simulink model "SF001A_Assi"  (R2013b)
settings: Solver=FixedStepDiscrete  StartTime=0.0  StopTime=1  FixedStep=.002  RelTol=1e-3
values from neighbouring files (symbols this model uses):
  FLTINJ_ASSI_ASSICMDBAS = DataDict.Constant    [SF001A_Assi_DataDict.m]
libraries: FixdToFloat x4, FloatToFixd x4, BilnrIntrpnMplX x3, NxtrLim x2, NxtrAbslt x1, NxtrMath x1, LnrIntrpn x1, NxtrSign x1, simulink x1
settings Model: Creator=lzz0tm  LastModifiedBy=HZQ8V7
settings DataIOCC: LimitDataPoints=off  SaveFormat=Structure  ReturnWorkspaceOutputs=on
settings OptimizationCC: BlockReduction=off  InlineParams=on  ZeroExternalMemoryAtStartup=off  ZeroInternalMemoryAtStartup=off  OptimizeModelRefInitCode=on  LifeSpan=1
settings DebuggingCC: SignalInfNanChecking=error  SignalRangeChecking=warning  UnderspecifiedInitializationDetection=Simplified  SolverPrmCheckMsg=error  InheritedTsInSrcMsg=error  DiscreteInheritContinuousMsg=error  SingleTaskRateTransMsg=error  TasksWithSamePriorityMsg=error  SigSpecEnsureSampleTimeMsg=error  CheckMatrixSingularityMsg=error  IntegerOverflowMsg=error  ParameterUnderflowMsg=error  ParameterPrecisionLossMsg=error  ParameterTunabilityLossMsg=error  FixptConstUnderflowMsg=warning  FixptConstOverflowMsg=warning  VectorMatrixConversionMsg=error  SignalLabelMismatchMsg=error  UnconnectedInputMsg=error  UnconnectedOutputMsg=error  UnconnectedLineMsg=error  SFcnCompatibilityMsg=error  UniqueDataStoreMsg=warning  BusObjectLabelMismatch=error  RootOutportRequireBusObject=error  AssertControl=DisableAll  ModelReferenceIOMsg=error  ModelReferenceVersionMismatchMessage=warning  ModelReferenceIOMismatchMessage=error  ModelReferenceCSMismatchMessage=warning  ModelReferenceDataLoggingMessage=error  StateNameClashWarn=warning  StrictBusMsg=ErrorOnBusTreatedAsVector  NonBusSignalsTreatedAsBus=error  SFUnexpectedBacktrackingDiag=error  SFInvalidInputDataAccessInChartInitDiag=error  SFNoUnconditionalDefaultTransitionDiag=error  SFTransitionOutsideNaturalParentDiag=error  SFUnconditionalTransitionShadowingDiag=error  SFUndirectedBroadcastEventsDiag=error
settings ModelReferenceCC: ModelReferenceNumInstancesAllowed=Single
settings RTWCC: SystemTargetFile=autosar.tlc  GenCodeOnly=on  TemplateMakefile=ert_default_tmf  Description=AUTOSAR  GenerateReport=on  ProcessScript=autosar_make_rtw_hook  LaunchReport=on
settings CodeAppCC: GenerateComments=off  IgnoreCustomStorageClasses=off  CustomSymbolStrType=$N$R$M  CustomSymbolStrBlkIO=$N$M  SimulinkBlockComments=off
settings STFCustomTargetCC: ParMdlRefBuildCompliant=on  CompOptLevelCompliant=on  IncludeMdlTerminateFcn=off  CombineOutputUpdateFcns=on  SuppressErrorStatus=on  ERTFirstTimeCompliant=on  ERTCustomFileBanners=on  SupportNonFinite=off  SupportComplex=off  SupportContinuousTime=off  SupportNonInlinedSFcns=off  MATLABClassNameForMDSCustomization=Simulink.SoftwareTarget.ERTCustomization  AutosarCompliant=on  GRTInterface=off  SystemTargetFile=autosar.tlc
settings ERTTargetCC: CodeReplacementLibrary=ANSI_C  ConcurrentExecutionCompliant=off  IncludeMdlTerminateFcn=off  SuppressErrorStatus=on  SupportNonFinite=off  SupportComplex=off  ModelStepFunctionPrototypeControlCompliant=off  CPPClassGenCompliant=off  AutosarCompliant=on  InlinedParameterPlacement=NonHierarchical  ERTCustomFileTemplate=example_file_process.tlc  EnableUserReplacementTypes=on

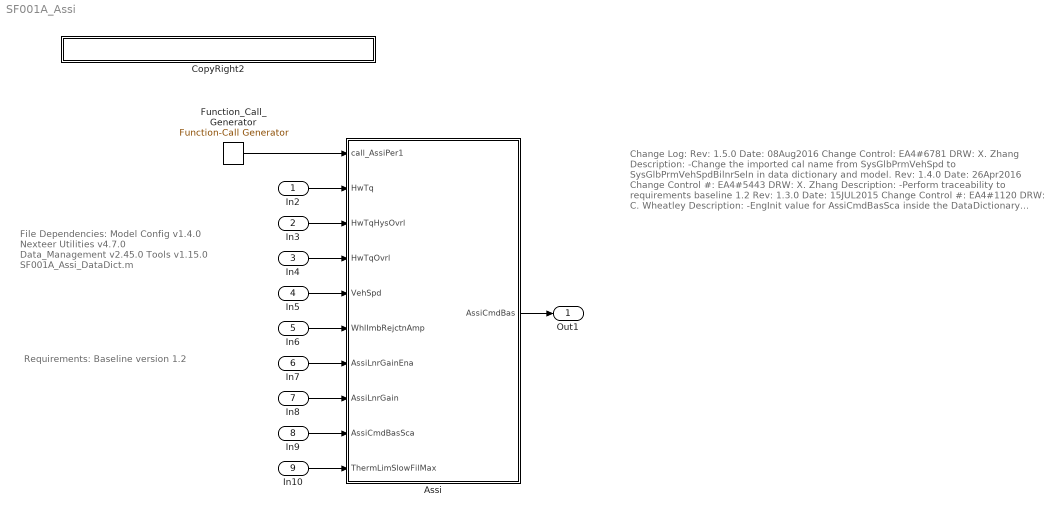
== system SF001A_Assi ==
  note: File Dependencies:
      |
      | Model Config v1.4.0
      | Nexteer Utilities v4.7.0
      | Data_Management v2.45.0
      | Tools v1.15.0
      | SF001A_Assi_DataDict.m
  note: Change Log:
      |
      | Rev: 1.5.0
      | Date: 08Aug2016
      | Change Control: EA4#6781
      | DRW: X. Zhang
      | Description:
      | -Change the imported cal name from SysGlbPrmVehSpd
      | to SysGlbPrmVehSpdBilnrSeln in data dictionary and model.
      |
      |
      | Rev: 1.4.0
      | Date: 26Apr2016
      | Change Control #: EA4#5443
      | DRW: X. Zhang
      | Description:
      | -Perform traceability to requirements baseline 1.2
      |
      | Rev: 1.3.0
      | Date: 15JUL2015
      | Change Control #: EA4#1120
      | DRW: C. Wheatley
      | Description:
      | -EngInit value for AssiCmdBasSca inside the
      |   DataDictionary changed to 1
      |
      | Rev: 1.2.0
      | Date: 09JUN2015
      | Change Control #: EA4#729
      | DRW: C. Wheatley
      | Description:
      | - Fault Injection mistake corrected in the model
      | - Variable names in DataDictionary changed to
      |    comply with AutoSar
      | - LongName and Description fixes in the
      |    DataDictionary
      | - Calibration settings corrected in DataDictionary
      | - Boolean If statement in model adjusted for
      |    readability
      | - Blend now using EA4 block
      | - Naming consistency in the model
      |
      | Rev: 1.1.0
      | Date: 28MAY2015
      | Change Control #: EA4#675
      | DRW: C. Wheatley
      | Description:
      | - Updated changes to the DataDictionary values
      | - Model updated to use global parameters
      |
      | Rev: 1.0.0
      | Date: 28APR2015
      | Change Control #: EA4#513
      | DRW: Wheatley
      | Description:
      | Initial EA4 Release
  note: Requirements: Baseline version 1.2
  In2 : Inport
  In3 : Inport  Port=2
  In4 : Inport  Port=3
  In5 : Inport  Port=4
  In6 : Inport  Port=5
  In7 : Inport  Port=6
  In8 : Inport  Port=7
  In9 : Inport  Port=8
  In10 : Inport  Port=9
  Assi : Subsystem
  CopyRight2 : Subsystem  Description=|  mask(Copyright Information){none=on}
      | Copyright info block.                                               
      |                                                                     
      | Place copyright information at the top of every subsystem in design.
      mask prompts: none "No parameters"
      mask help: Place copyright information at the top of every subsystem in design.
      mask Display:
      | NxtrConf = 'Nexteer Confidential';
      | 
      | sys = bdroot; %handle for the current model ("system")
      | first = get_param(sys,'Created');
      | first = first(end-3:end);  %year is last four digits
      | 
      | last = get_param(sys,'LastModifiedDate');
      | if isempty(last)
      |     last = datestr(now,'yyyy');
      | else
      |     last = last(end-3:end);
      | end
      | 
      | if strcmp(first,last)
      |     fprintf('%s -- Copyright %s Nexteer',NxtrConf,first)
      | else
      |     fprintf('%s -- %s%s- %s Nexteer',NxtrConf,char(169),first,last)
      | end
  Function_Call_Generator : simulink/Ports & Subsystems/Function-Call Generator  sample_time=1  numberOfIterations=1
  Out1 : Outport
  wires:
  In4/1 -> Assi/4(HwTqOvrl)
  In3/1 -> Assi/3(HwTqHysOvrl)
  In2/1 -> Assi/2(HwTq)
  Function_Call_Generator/1 -> Assi/1("call_AssiPer1 ")
  In5/1 -> Assi/5(VehSpd)
  In6/1 -> Assi/6(WhlImbRejctnAmp)
  In7/1 -> Assi/7(AssiLnrGainEna)
  In8/1 -> Assi/8(AssiLnrGain)
  In9/1 -> Assi/9(AssiCmdBasSca)
  In10/1 -> Assi/10(ThermLimSlowFilMax)
  Assi/1(AssiCmdBas) -> Out1/1

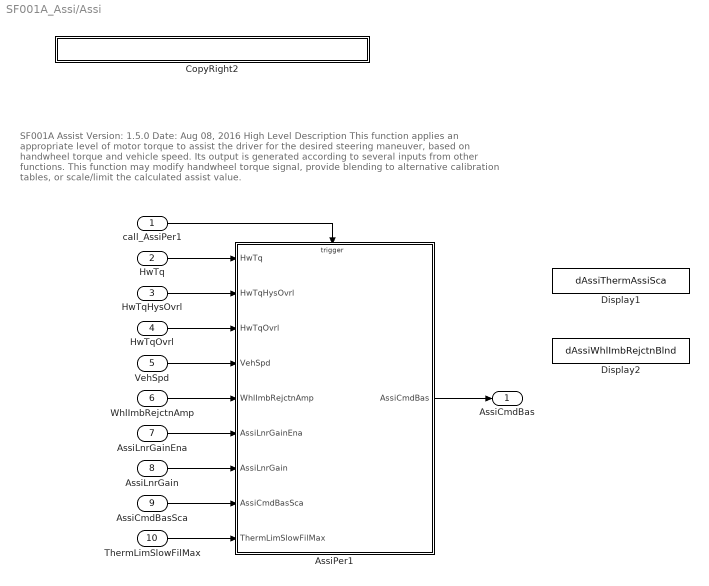
== system SF001A_Assi/Assi ==
  note: SF001A Assist                                                                                  Version:  1.5.0         Date:  Aug 08, 2016
      |  High Level Description
      |
      | This function applies an appropriate level of motor torque to assist the driver for the desired steering maneuver,
      | based on handwheel torque and vehicle speed. Its output is generated according to several inputs from other functions.
      | This function may modify handwheel torque signal, provide blending to alternative calibration tables, or scale/limit the calculated assist value.
  "call_AssiPer1 " : Inport
  HwTq : Inport  RequirementInfo={'linktype_rmi_doors' '0000a523 (/E-STEER Core/SubSystem Specifications/Application Functions/SF001A Assist)' '#SF001A_565' 'true' 'REQ: SF001A_565' '' } %GIDa_df1c7e41_35b1_4231_b879_3ebd4c9f1c76  Port=2  PortDimensions=1
  HwTqHysOvrl : Inport  RequirementInfo={'linktype_rmi_doors' '0000a523 (/E-STEER Core/SubSystem Specifications/Application Functions/SF001A Assist)' '#SF001A_566' 'true' 'REQ: SF001A_566' '' } %GIDa_321f90ce_d978_4ab3_928c_b38d2719cd45  Port=3
  HwTqOvrl : Inport  RequirementInfo={'linktype_rmi_doors' '0000a523 (/E-STEER Core/SubSystem Specifications/Application Functions/SF001A Assist)' '#SF001A_566' 'true' 'REQ: SF001A_566' '' } %GIDa_7605816b_6934_4ac2_b90b_cbcd1f03215b  Port=4
  VehSpd : Inport  RequirementInfo={'linktype_rmi_doors' '0000a523 (/E-STEER Core/SubSystem Specifications/Application Functions/SF001A Assist)' '#SF001A_566' 'true' 'REQ: SF001A_566' '' } %GIDa_a7343de8_f548_4ff5_81a9_3f5168f89c4e  Port=5
  WhlImbRejctnAmp : Inport  RequirementInfo={'linktype_rmi_doors' '0000a523 (/E-STEER Core/SubSystem Specifications/Application Functions/SF001A Assist)' '#SF001A_569' 'true' 'REQ: SF001A_569' '' } %GIDa_b330648f_a269_46fd_8bc1_16a6ad0b258f  Port=6
  AssiLnrGainEna : Inport  RequirementInfo={'linktype_rmi_doors' '0000a523 (/E-STEER Core/SubSystem Specifications/Application Functions/SF001A Assist)' '#SF001A_570' 'true' 'REQ: SF001A_570' '' } %GIDa_c83e3dc0_0b95_4f73_8c8d_f554ad8bd146  Port=7
  AssiLnrGain : Inport  RequirementInfo={'linktype_rmi_doors' '0000a523 (/E-STEER Core/SubSystem Specifications/Application Functions/SF001A Assist)' '#SF001A_571' 'true' 'REQ: SF001A_571' '' } %GIDa_7839c29a_d675_4409_929b_04df3bfe5379  Port=8
  AssiCmdBasSca : Inport  RequirementInfo={'linktype_rmi_doors' '0000a523 (/E-STEER Core/SubSystem Specifications/Application Functions/SF001A Assist)' '#SF001A_572' 'true' 'REQ: SF001A_572' '' } %GIDa_8964cba7_7b16_46dc_9776_5743dbedca3e  Port=9
  ThermLimSlowFilMax : Inport  RequirementInfo={'linktype_rmi_doors' '0000a523 (/E-STEER Core/SubSystem Specifications/Application Functions/SF001A Assist)' '#SF001A_573' 'true' 'REQ: SF001A_573' '' } %GIDa_45ade21b_63ba_460c_b3cc_31c25871d07a  Port=10
  AssiPer1 : Subsystem
  CopyRight2 : Subsystem  Description=|  mask(Copyright Information){none=on}
      | Copyright info block.                                               
      |                                                                     
      | Place copyright information at the top of every subsystem in design.
      mask prompts: none "No parameters"
      mask help: Place copyright information at the top of every subsystem in design.
      mask Display:
      | NxtrConf = 'Nexteer Confidential';
      | 
      | sys = bdroot; %handle for the current model ("system")
      | first = get_param(sys,'Created');
      | first = first(end-3:end);  %year is last four digits
      | 
      | last = get_param(sys,'LastModifiedDate');
      | if isempty(last)
      |     last = datestr(now,'yyyy');
      | else
      |     last = last(end-3:end);
      | end
      | 
      | if strcmp(first,last)
      |     fprintf('%s -- Copyright %s Nexteer',NxtrConf,first)
      | else
      |     fprintf('%s -- %s%s- %s Nexteer',NxtrConf,char(169),first,last)
      | end
  Display1 : DataStoreMemory  DataStoreName=dAssiThermAssiSca  ReadBeforeWriteMsg=warning  WriteAfterWriteMsg=warning  WriteAfterReadMsg=warning  StateMustResolveToSignalObject=on
  Display2 : DataStoreMemory  DataStoreName=dAssiWhlImbRejctnBlnd  ReadBeforeWriteMsg=warning  WriteAfterWriteMsg=warning  WriteAfterReadMsg=warning  StateMustResolveToSignalObject=on
  AssiCmdBas : Outport  RequirementInfo={'linktype_rmi_doors' '0000a523 (/E-STEER Core/SubSystem Specifications/Application Functions/SF001A Assist)' '#SF001A_573' 'true' 'REQ: SF001A_573' '' } %GIDa_c295ac1d_a023_4c71_a7e9_db668cfce82d
  wires:
  "call_AssiPer1 "/1 -> AssiPer1/Trigger
  AssiCmdBasSca/1 -> AssiPer1/8(AssiCmdBasSca)
  ThermLimSlowFilMax/1 -> AssiPer1/9(ThermLimSlowFilMax)
  HwTqOvrl/1 -> AssiPer1/3(HwTqOvrl)
  HwTqHysOvrl/1 -> AssiPer1/2(HwTqHysOvrl)
  HwTq/1 -> AssiPer1/1(HwTq)
  AssiLnrGain/1 -> AssiPer1/7(AssiLnrGain)
  WhlImbRejctnAmp/1 -> AssiPer1/5(WhlImbRejctnAmp)
  AssiPer1/1(AssiCmdBas) -> AssiCmdBas/1
  AssiLnrGainEna/1 -> AssiPer1/6(AssiLnrGainEna)
  VehSpd/1 -> AssiPer1/4(VehSpd)

== system SF001A_Assi/CopyRight2 ==

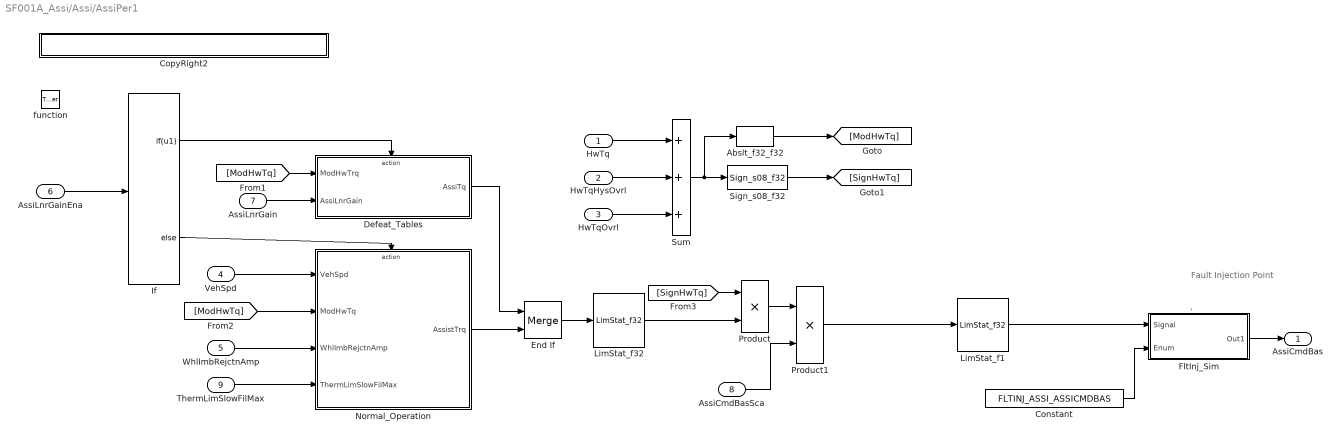
== system SF001A_Assi/Assi/AssiPer1 ==
  note: ,
  note: Fault
      | Injection
      | Point
  HwTq : Inport  RequirementInfo={'linktype_rmi_doors' '0000a523 (/E-STEER Core/SubSystem Specifications/Application Functions/SF001A Assist)' '#SF001A_565' 'true' 'REQ: SF001A_565' '' } %GIDa_4c532047_88a3_4a73_b7dd_64dbcaaed348  PortDimensions=1
  HwTqHysOvrl : Inport  RequirementInfo={'linktype_rmi_doors' '0000a523 (/E-STEER Core/SubSystem Specifications/Application Functions/SF001A Assist)' '#SF001A_565' 'true' 'REQ: SF001A_565' '' } %GIDa_a6de7906_5536_4fc7_b71a_7e4fd7338639  Port=2
  HwTqOvrl : Inport  RequirementInfo={'linktype_rmi_doors' '0000a523 (/E-STEER Core/SubSystem Specifications/Application Functions/SF001A Assist)' '#SF001A_565' 'true' 'REQ: SF001A_565' '' } %GIDa_743579df_9034_4b45_9394_2ab6ce07898f  Port=3
  VehSpd : Inport  Port=4
  WhlImbRejctnAmp : Inport  Port=5
  AssiLnrGainEna : Inport  Port=6
  AssiLnrGain : Inport  Port=7
  AssiCmdBasSca : Inport  RequirementInfo={'linktype_rmi_doors' '0000a523 (/E-STEER Core/SubSystem Specifications/Application Functions/SF001A Assist)' '#SF001A_54' 'true' 'REQ: SF001A_54' '' } %GIDa_4f99cdde_4310_4043_a572_c6e40ed4e5b1  Port=8
  ThermLimSlowFilMax : Inport  Port=9
  function : TriggerPort  TriggerType=function-call  PortDimensions=1
  Abslt_f32_f32 : NxtrAbslt/Abslt_f32_f32  RequirementInfo={'linktype_rmi_doors' '0000a523 (/E-STEER Core/SubSystem Specifications/Application Functions/SF001A Assist)' '#SF001A_565' 'true' 'REQ: SF001A_565' '' } %GIDa_e7f45768_8990_4d11_92fe_2addd2fec813  SFunctionSpec=single y1 = Abslt_f32_f32(single u1)
  Constant : Constant  Value=FLTINJ_ASSI_ASSICMDBAS
  CopyRight2 : Subsystem  Description=|  mask(Copyright Information){none=on}
      | Copyright info block.                                               
      |                                                                     
      | Place copyright information at the top of every subsystem in design.
      mask prompts: none "No parameters"
      mask help: Place copyright information at the top of every subsystem in design.
      mask Display:
      | NxtrConf = 'Nexteer Confidential';
      | 
      | sys = bdroot; %handle for the current model ("system")
      | first = get_param(sys,'Created');
      | first = first(end-3:end);  %year is last four digits
      | 
      | last = get_param(sys,'LastModifiedDate');
      | if isempty(last)
      |     last = datestr(now,'yyyy');
      | else
      |     last = last(end-3:end);
      | end
      | 
      | if strcmp(first,last)
      |     fprintf('%s -- Copyright %s Nexteer',NxtrConf,first)
      | else
      |     fprintf('%s -- %s%s- %s Nexteer',NxtrConf,char(169),first,last)
      | end
  Defeat_Tables : Subsystem  RequirementInfo={} %GIDa_71bd2140_2601_481a_a962_dd66954b4836  TreatAsAtomicUnit=on
  End If : Merge
  FltInj_Sim : Subsystem  RequirementInfo={} %GIDa_e6d32a6b_110d_43d3_bf1f_53358b823df8  TreatAsAtomicUnit=on  VariantControl=FltInj_sim  mask(Fault_Injection){}
      mask help: Fault Injection is a simulation only block for EA4 programs.
  If : If  RequirementInfo={'linktype_rmi_doors' '0000a523 (/E-STEER Core/SubSystem Specifications/Application Functions/SF001A Assist)' '#SF001A_584' 'true' 'REQ: SF001A_584' '' ; 'linktype_rmi_doors' '0000a523 (/E-STEER Core/SubSystem Specifications/Application Functions/SF001A Assist)' '#SF001A_586' 'true' 'REQ: SF001A_586' '' } %GIDa_38834bf7_fb6d_4a7f_939f_eb78c484652c  IfExpression=u1
  LimStat_f1 : NxtrLim/LimStat_f32  RequirementInfo={'linktype_rmi_doors' '0000a523 (/E-STEER Core/SubSystem Specifications/Application Functions/SF001A Assist)' '#SF001A_596' 'true' 'REQ: SF001A_596' '' } %GIDa_3652e6d3_c985_43e4_abfc_04d6d52d1687  LoLim=SYSGLBPRM_MOTTQCMDLOLIM_MOTNWTMTR_F32  HiLim=SYSGLBPRM_MOTTQCMDHILIM_MOTNWTMTR_F32
      settings: AttributesFormatString=|
      | Low Limit: %<LoLim>
      | High Limit: %<HiLim>
  LimStat_f32 : NxtrLim/LimStat_f32  RequirementInfo={'linktype_rmi_doors' '0000a523 (/E-STEER Core/SubSystem Specifications/Application Functions/SF001A Assist)' '#SF001A_593' 'true' 'REQ: SF001A_593' '' } %GIDa_e2683ff8_6aed_4c9d_9aec_fac7f0f7d52d  LoLim=ASSITQSFTYLIM_MOTNWTMTR_F32  HiLim=SYSGLBPRM_MOTTQCMDHILIM_MOTNWTMTR_F32
      settings: AttributesFormatString=|
      | Low Limit: %<LoLim>
      | High Limit: %<HiLim>
  Normal_Operation : Subsystem  RequirementInfo={} %GIDa_a17e3b27_231d_4f75_8813_4f769b98bbc6  TreatAsAtomicUnit=on
  Product : Product  RequirementInfo={'linktype_rmi_doors' '0000a523 (/E-STEER Core/SubSystem Specifications/Application Functions/SF001A Assist)' '#SF001A_595' 'true' 'REQ: SF001A_595' '' } %GIDa_1e6d8c6c_cd19_4240_97f1_349498f31d5f  RndMeth=Zero
  Product1 : Product  RequirementInfo={'linktype_rmi_doors' '0000a523 (/E-STEER Core/SubSystem Specifications/Application Functions/SF001A Assist)' '#SF001A_595' 'true' 'REQ: SF001A_595' '' } %GIDa_d1996e46_02c0_494a_8107_cfbf4a1e6ec3  RndMeth=Zero
  Sign_s08_f32 : NxtrSign/Sign_s08_f32  RequirementInfo={} %GIDa_76fc9d16_9ca3_42b5_94b3_bead8e1e389b  SFunctionSpec=int8 y1 = Sign_s08_f32(single u1)
  Sum : Sum  RequirementInfo={'linktype_rmi_doors' '0000a523 (/E-STEER Core/SubSystem Specifications/Application Functions/SF001A Assist)' '#SF001A_581' 'true' 'REQ: SF001A_581' '' } %GIDa_5bf640b0_a2a0_4a1b_859a_3210dc25e735  Inputs=+++
  AssiCmdBas : Outport  RequirementInfo={} %GIDa_2c9965c4_fb6f_4fb8_804f_ca6f7a7ece36
  wires:
  Product1/1 -> LimStat_f1/1
  Abslt_f32_f32/1 -> [ModHwTq]
  [SignHwTq] -> Product/1
  Sum/1 -> Sign_s08_f32/1, Abslt_f32_f32/1
  HwTq/1 -> Sum/1
  HwTqHysOvrl/1 -> Sum/2
  HwTqOvrl/1 -> Sum/3
  AssiLnrGainEna/1 -> If/1
  If/1 -> Defeat_Tables/Action
  If/2 -> Normal_Operation/Action
  [ModHwTq] -> Defeat_Tables/1(ModHwTrq)
  [ModHwTq] -> Normal_Operation/2(ModHwTq)
  WhlImbRejctnAmp/1 -> Normal_Operation/3(WhlImbRejctnAmp)
  VehSpd/1 -> Normal_Operation/1(VehSpd)
  Defeat_Tables/1(AssiTq) -> End If/1
  Normal_Operation/1(AssistTrq) -> End If/2
  AssiLnrGain/1 -> Defeat_Tables/2(AssiLnrGain)
  Product/1 -> Product1/1
  ThermLimSlowFilMax/1 -> Normal_Operation/4(ThermLimSlowFilMax)
  AssiCmdBasSca/1 -> Product1/2
  Sign_s08_f32/1 -> [SignHwTq]
  End If/1 -> LimStat_f32/1
  LimStat_f32/1 -> Product/2
  LimStat_f1/1 -> FltInj_Sim/1(Signal)
  Constant/1 -> FltInj_Sim/2(Enum)
  FltInj_Sim/1(Out1) -> AssiCmdBas/1

== system SF001A_Assi/Assi/CopyRight2 ==

== system SF001A_Assi/Assi/AssiPer1/CopyRight2 ==

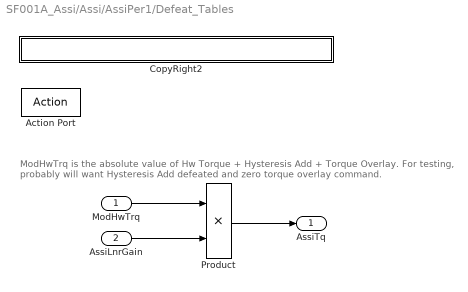
== system SF001A_Assi/Assi/AssiPer1/Defeat_Tables ==
  note: ModHwTrq is the absolute value of Hw Torque  +  Hysteresis Add  +  Torque Overlay.
      | For testing, probably will want Hysteresis Add defeated and zero torque overlay command.
  ModHwTrq : Inport
  AssiLnrGain : Inport  Port=2
  Action Port : ActionPort  ActionType=then
  CopyRight2 : Subsystem  Description=|  mask(Copyright Information){none=on}
      | Copyright info block.                                               
      |                                                                     
      | Place copyright information at the top of every subsystem in design.
      mask prompts: none "No parameters"
      mask help: Place copyright information at the top of every subsystem in design.
      mask Display:
      | NxtrConf = 'Nexteer Confidential';
      | 
      | sys = bdroot; %handle for the current model ("system")
      | first = get_param(sys,'Created');
      | first = first(end-3:end);  %year is last four digits
      | 
      | last = get_param(sys,'LastModifiedDate');
      | if isempty(last)
      |     last = datestr(now,'yyyy');
      | else
      |     last = last(end-3:end);
      | end
      | 
      | if strcmp(first,last)
      |     fprintf('%s -- Copyright %s Nexteer',NxtrConf,first)
      | else
      |     fprintf('%s -- %s%s- %s Nexteer',NxtrConf,char(169),first,last)
      | end
  Product : Product  RequirementInfo={} %GIDa_47c2f9d0_cfe8_45f5_bf6e_658d390a0821  RndMeth=Zero
  AssiTq : Outport  RequirementInfo={'linktype_rmi_doors' '0000a523 (/E-STEER Core/SubSystem Specifications/Application Functions/SF001A Assist)' '#SF001A_585' 'true' 'REQ: SF001A_585' '' } %GIDa_b2d1d4b3_a613_4d35_bc31_c1b4db410c70
  wires:
  ModHwTrq/1 -> Product/1
  Product/1 -> AssiTq/1
  AssiLnrGain/1 -> Product/2

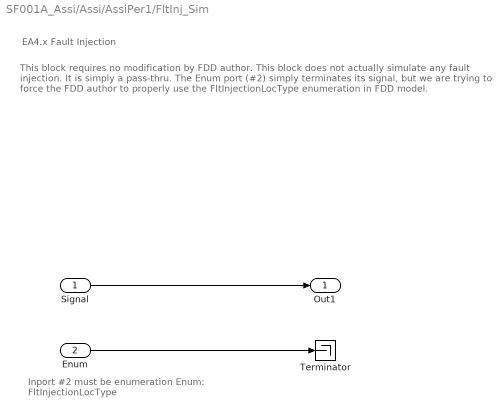
== system SF001A_Assi/Assi/AssiPer1/FltInj_Sim ==
  note: Inport #2 must be enumeration
      | Enum: FltInjectionLocType
  note: EA4.x Fault Injection
  note: This block requires no modification by FDD author.
      |
      | This block does not actually simulate any fault injection.  It is simply a pass-thru.
      |
      | The Enum port (#2) simply terminates its signal, but we are trying to force the FDD author
      | to properly use the FltInjectionLocType enumeration in FDD model.
  Signal : Inport
  Enum : Inport  Port=2
  Terminator : Terminator
  Out1 : Outport
  wires:
  Enum/1 -> Terminator/1
  Signal/1 -> Out1/1

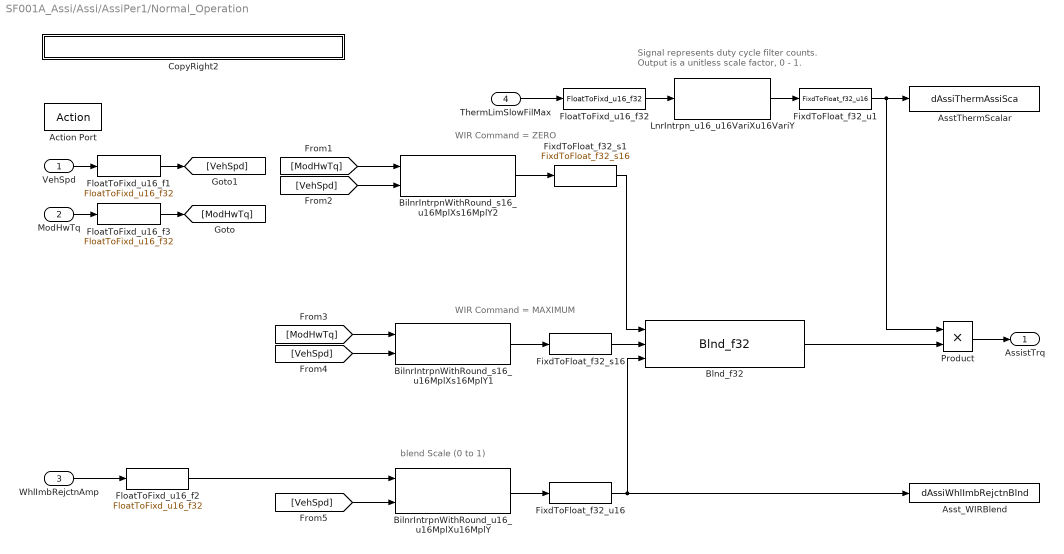
== system SF001A_Assi/Assi/AssiPer1/Normal_Operation ==
  note: blend Scale (0 to 1)
  note: WIR Command = ZERO
  note: WIR Command = MAXIMUM
  note: Signal represents duty cycle filter counts.
      | Output is a unitless scale factor, 0 - 1.
  VehSpd : Inport
  ModHwTq : Inport  Port=2
  WhlImbRejctnAmp : Inport  Port=3
  ThermLimSlowFilMax : Inport  RequirementInfo={'linktype_rmi_doors' '0000a523 (/E-STEER Core/SubSystem Specifications/Application Functions/SF001A Assist)' '#SF001A_53' 'true' 'REQ: SF001A_53' '' } %GIDa_d495ecea_f09d_4663_8f43_a6d971893cb5  Port=4
  Action Port : ActionPort  ActionType=else
  AsstThermScalar : DataStoreWrite  RequirementInfo={'linktype_rmi_doors' '0000a523 (/E-STEER Core/SubSystem Specifications/Application Functions/SF001A Assist)' '#SF001A_53' 'true' 'REQ: SF001A_53' '' } %GIDa_cc140d46_460a_48ba_8b3e_79cf1600f1e9  DataStoreName=dAssiThermAssiSca
  Asst_WIRBlend : DataStoreWrite  RequirementInfo={'linktype_rmi_doors' '0000a523 (/E-STEER Core/SubSystem Specifications/Application Functions/SF001A Assist)' '#SF001A_52' 'true' 'REQ: SF001A_52' '' } %GIDa_adaeb4d5_68f1_4d88_ac20_3bce34d2e10b  DataStoreName=dAssiWhlImbRejctnBlnd
  BilnrIntrpnWithRound_s16_u16MplXs16MplY1 : BilnrIntrpnMplX/BilnrIntrpnWithRound_s16_u16MplXs16MplY  RequirementInfo={'linktype_rmi_doors' '0000a523 (/E-STEER Core/SubSystem Specifications/Application Functions/SF001A Assist)' '#SF001A_588' 'true' 'REQ: SF001A_588' '' } %GIDa_8cd23924_1daf_4ef2_bbb5_07ceb7e349f6  MplXTbl=AssiMotTqWhlImbRejctnMaxX  MplYTbl=AssiMotTqWhlImbRejctnMaxY  BilnrSelnTbl=SysGlbPrmVehSpdBilnrSeln
      settings: AttributesFormatString=|
      | Bilnr ( u16MplX , s16MplY )
      | XTbl: %<MplXTbl>
      | YTbl: %<MplYTbl>
      | BilnrSelnTbl: %<BilnrSelnTbl>
  BilnrIntrpnWithRound_s16_u16MplXs16MplY2 : BilnrIntrpnMplX/BilnrIntrpnWithRound_s16_u16MplXs16MplY  RequirementInfo={'linktype_rmi_doors' '0000a523 (/E-STEER Core/SubSystem Specifications/Application Functions/SF001A Assist)' '#SF001A_587' 'true' 'REQ: SF001A_587' '' } %GIDa_029eacd6_36ad_4f40_9925_dba968d6273e  MplXTbl=AssiMotTqWhlImbRejctnMinX  MplYTbl=AssiMotTqWhlImbRejctnMinY  BilnrSelnTbl=SysGlbPrmVehSpdBilnrSeln
      settings: AttributesFormatString=|
      | Bilnr ( u16MplX , s16MplY )
      | XTbl: %<MplXTbl>
      | YTbl: %<MplYTbl>
      | BilnrSelnTbl: %<BilnrSelnTbl>
  BilnrIntrpnWithRound_u16_u16MplXu16MplY : BilnrIntrpnMplX/BilnrIntrpnWithRound_u16_u16MplXu16MplY  RequirementInfo={'linktype_rmi_doors' '0000a523 (/E-STEER Core/SubSystem Specifications/Application Functions/SF001A Assist)' '#SF001A_589' 'true' 'REQ: SF001A_589' '' } %GIDa_7c428585_68bf_4d65_87df_925e8b40f134  MplXTbl=AssiWhlImbRejctnBlndScaX  MplYTbl=AssiWhlImbRejctnBlndScaY  BilnrSelnTbl=SysGlbPrmVehSpdBilnrSeln
      settings: AttributesFormatString=|
      | Bilnr ( u16MplX , u16MplY )
      | XTbl: %<MplXTbl>
      | YTbl: %<MplYTbl>
      | BilnrSelnTbl: %<BilnrSelnTbl>
  Blnd_f32 : NxtrMath/Blnd_f32  RequirementInfo={'linktype_rmi_doors' '0000a523 (/E-STEER Core/SubSystem Specifications/Application Functions/SF001A Assist)' '#SF001A_590' 'true' 'REQ: SF001A_590' '' } %GIDa_cff7a165_44c8_4e31_be82_33768175da9d  SFunctionSpec=single y1 = Blnd_f32(single u1, single u2, single u3)  Parameter3=on
      settings: AttributesFormatString=%<Name>
  CopyRight2 : Subsystem  Description=|  mask(Copyright Information){none=on}
      | Copyright info block.                                               
      |                                                                     
      | Place copyright information at the top of every subsystem in design.
      mask prompts: none "No parameters"
      mask help: Place copyright information at the top of every subsystem in design.
      mask Display:
      | NxtrConf = 'Nexteer Confidential';
      | 
      | sys = bdroot; %handle for the current model ("system")
      | first = get_param(sys,'Created');
      | first = first(end-3:end);  %year is last four digits
      | 
      | last = get_param(sys,'LastModifiedDate');
      | if isempty(last)
      |     last = datestr(now,'yyyy');
      | else
      |     last = last(end-3:end);
      | end
      | 
      | if strcmp(first,last)
      |     fprintf('%s -- Copyright %s Nexteer',NxtrConf,first)
      | else
      |     fprintf('%s -- %s%s- %s Nexteer',NxtrConf,char(169),first,last)
      | end
  FixdToFloat_f32_s1 : FixdToFloat/FixdToFloat_f32_s16  Param1=11
  FixdToFloat_f32_s16 : FixdToFloat/FixdToFloat_f32_s16  Param1=11
  FixdToFloat_f32_u1 : FixdToFloat/FixdToFloat_f32_u16  Param1=14
  FixdToFloat_f32_u16 : FixdToFloat/FixdToFloat_f32_u16  Param1=14
  FloatToFixd_u16_f1 : FloatToFixd/FloatToFixd_u16_f32  Param1=7
  FloatToFixd_u16_f2 : FloatToFixd/FloatToFixd_u16_f32  Param1=11
  FloatToFixd_u16_f3 : FloatToFixd/FloatToFixd_u16_f32  Param1=8
  FloatToFixd_u16_f32 : FloatToFixd/FloatToFixd_u16_f32  Param1=single(0)
  LnrIntrpn_u16_u16VariXu16VariY : LnrIntrpn/LnrIntrpn_u16_u16VariXu16VariY  RequirementInfo={} %GIDa_0cb1498c_b9e2_4aae_adbb_780c9161840b  XTbl=AssiThermScaX  YTbl=AssiThermScaY
      settings: AttributesFormatString=|
      | Lnr ( u16VariX , u16VariY )
      | XTbl: %<XTbl>
      | YTbl: %<YTbl>
  Product : Product  RequirementInfo={} %GIDa_8efe5603_90ed_4642_a016_f9c1166e0ef2  RndMeth=Zero
  AssistTrq : Outport  RequirementInfo={'linktype_rmi_doors' '0000a523 (/E-STEER Core/SubSystem Specifications/Application Functions/SF001A Assist)' '#SF001A_591' 'true' 'REQ: SF001A_591' '' } %GIDa_02181a13_0e68_41db_a2f9_656623ee604d
  wires:
  BilnrIntrpnWithRound_u16_u16MplXu16MplY/1 -> FixdToFloat_f32_u16/1
  BilnrIntrpnWithRound_s16_u16MplXs16MplY2/1 -> FixdToFloat_f32_s1/1
  Blnd_f32/1 -> Product/2
  Product/1 -> AssistTrq/1
  FixdToFloat_f32_s1/1 -> Blnd_f32/1
  FixdToFloat_f32_u16/1 -> Asst_WIRBlend/1, Blnd_f32/3
  WhlImbRejctnAmp/1 -> FloatToFixd_u16_f2/1
  [VehSpd] -> BilnrIntrpnWithRound_u16_u16MplXu16MplY/2
  [VehSpd] -> BilnrIntrpnWithRound_s16_u16MplXs16MplY1/2
  [VehSpd] -> BilnrIntrpnWithRound_s16_u16MplXs16MplY2/2
  FixdToFloat_f32_s16/1 -> Blnd_f32/2
  BilnrIntrpnWithRound_s16_u16MplXs16MplY1/1 -> FixdToFloat_f32_s16/1
  VehSpd/1 -> FloatToFixd_u16_f1/1
  FloatToFixd_u16_f3/1 -> [ModHwTq]
  ModHwTq/1 -> FloatToFixd_u16_f3/1
  [ModHwTq] -> BilnrIntrpnWithRound_s16_u16MplXs16MplY2/1
  [ModHwTq] -> BilnrIntrpnWithRound_s16_u16MplXs16MplY1/1
  ThermLimSlowFilMax/1 -> FloatToFixd_u16_f32/1
  FloatToFixd_u16_f32/1 -> LnrIntrpn_u16_u16VariXu16VariY/1
  FixdToFloat_f32_u1/1 -> Product/1, AsstThermScalar/1
  LnrIntrpn_u16_u16VariXu16VariY/1 -> FixdToFloat_f32_u1/1
  FloatToFixd_u16_f1/1 -> [VehSpd]
  FloatToFixd_u16_f2/1 -> BilnrIntrpnWithRound_u16_u16MplXu16MplY/1

== system SF001A_Assi/Assi/AssiPer1/Defeat_Tables/CopyRight2 ==

== system SF001A_Assi/Assi/AssiPer1/Normal_Operation/CopyRight2 ==
